simulink subsystem "data_logging_for_ego_veh_subsystem"  (R2025a)
settings: Solver=VariableStepAuto  StartTime=0.0  StopTime=10.0  RelTol=1e-3
settings Model: Creator=admin  LastModifiedBy=admin

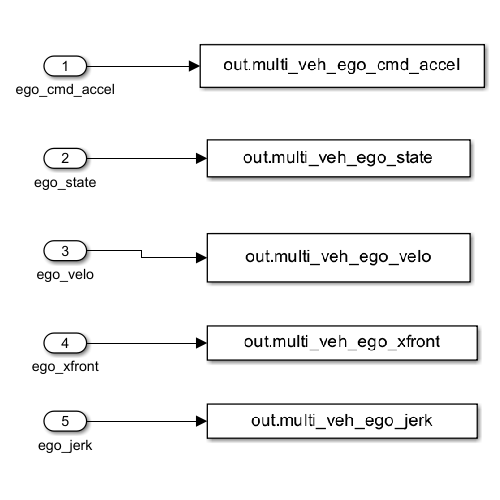
[thumbnail: Simulink's stored preview of the top-level diagram]
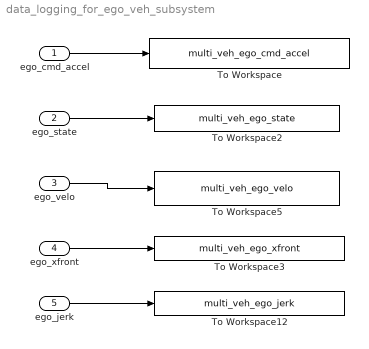
== system data_logging_for_ego_veh_subsystem ==
  ego_cmd_accel : Inport
  ego_state : Inport  Port=2
  ego_velo : Inport  Port=3
  ego_xfront : Inport  Port=4
  ego_jerk : Inport  Port=5
  To Workspace : ToWorkspace  VariableName=multi_veh_ego_cmd_accel  SaveFormat=Structure With Time  SampleTime=-1
  To Workspace12 : ToWorkspace  VariableName=multi_veh_ego_jerk  SaveFormat=Structure With Time  SampleTime=-1
  To Workspace2 : ToWorkspace  VariableName=multi_veh_ego_state  SaveFormat=Structure With Time  SampleTime=-1
  To Workspace3 : ToWorkspace  VariableName=multi_veh_ego_xfront  SaveFormat=Structure With Time  SampleTime=-1
  To Workspace5 : ToWorkspace  VariableName=multi_veh_ego_velo  SaveFormat=Structure With Time  SampleTime=-1
  wires:
  ego_state/1 -> To Workspace2/1
  ego_xfront/1 -> To Workspace3/1
  ego_jerk/1 -> To Workspace12/1
  ego_cmd_accel/1 -> To Workspace/1
  ego_velo/1 -> To Workspace5/1
